simulink model "pendcart_temp"  (Simulink 8.9)
settings: Solver=ode45  StartTime=0.0  StopTime=tsim  RelTol=1e-3  EnableMultiTasking=on
values from neighbouring files (symbols this model uses):
  b = 0.01    [pendcartsim.m]
  c = 0.05    [pendcartsim.m]
  Eta = 0.5882    [pendcartsim.m]
  g = 9.82    [pendcartsim.m]
  K = 0.1    [pendcartsim.m]
  K1 = -119.0071    [pendcartsim.m]
  K2 = 0.0402    [pendcartsim.m]
  l = 0.5    [pendcartsim.m]
  L = 0.001    [pendcartsim.m]
  M = 1    [pendcartsim.m]
  m = 0.5    [pendcartsim.m]
  N = 50    [pendcartsim.m]
  p = 5.4277    [pendcartsim.m]
  p1 = 25.4277    [pendcartsim.m]
  R = 0.6575    [pendcartsim.m]
  theta0 = 5*pi/180    (= 0.0872664625997)    [pendcartsim.m]
  Wheel_Radius = 0.035    [pendcartsim.m]
undefined symbols (not defined in the file or in its folder): Taum, taum
settings Model: Creator=Chris  LastModifiedBy=Administrator
settings OptimizationCC: ExpressionDepthLimit=2147483647  InitFltsAndDblsToZero=on
settings DebuggingCC: AlgebraicLoopMsg=none  SaveWithParameterizedLinksMsg=none
settings GRTTargetCC: TargetFcnLib=ansi_tfl_tmw.mat

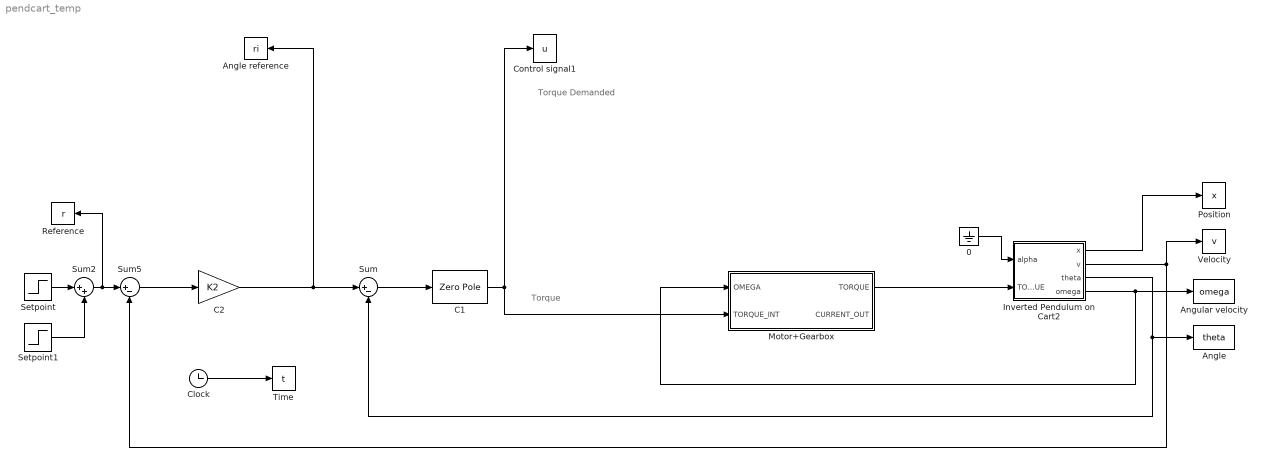
== system pendcart_temp ==
  note: Torque
  note: Torque Demanded
  0 : Ground
  Angle : ToWorkspace  VariableName=theta  SampleTime=-1
  Angle reference : ToWorkspace  VariableName=ri  SampleTime=-1
  Angular velocity : ToWorkspace  VariableName=omega  SampleTime=-1
  C1 : ZeroPole  Zeros=[-p]  Poles=[-p1]  Gain=[K1]
  C2 : Gain  Gain=K2
  Clock : Clock
  Control signal1 : ToWorkspace  VariableName=u  SampleTime=-1
  Inverted Pendulum on Cart2 : Subsystem
  Motor+Gearbox : Subsystem
  Position : ToWorkspace  VariableName=x  SampleTime=-1
  Reference : ToWorkspace  VariableName=r  SampleTime=-1
  Setpoint : Step  Time=10  After=0.5  SampleTime=0
  Setpoint1 : Step  Time=20  After=-0.5  SampleTime=0
  Sum : Sum  Inputs=|+-
  Sum2 : Sum  Inputs=|++
  Sum5 : Sum  Inputs=|+-
  Time : ToWorkspace  VariableName=t  SampleTime=-1
  Velocity : ToWorkspace  VariableName=v  SampleTime=-1
  wires:
  Clock/1 -> Time/1
  Inverted Pendulum on Cart2/1(x) -> Position/1
  Sum/1 -> C1/1
  C1/1 -> Motor+Gearbox/2(TORQUE_INT), Control signal1/1
  Inverted Pendulum on Cart2/2(v) -> Sum5/2, Velocity/1
  Inverted Pendulum on Cart2/3(theta) -> Sum/2, Angle/1
  Sum5/1 -> C2/1
  C2/1 -> Angle reference/1, Sum/1
  Setpoint/1 -> Sum2/1
  Setpoint1/1 -> Sum2/2
  Sum2/1 -> Sum5/1, Reference/1
  0/1 -> Inverted Pendulum on Cart2/1(alpha)
  Inverted Pendulum on Cart2/4(omega) -> Motor+Gearbox/1(OMEGA), Angular velocity/1
  Motor+Gearbox/1(TORQUE) -> Inverted Pendulum on Cart2/2(TORQUE)

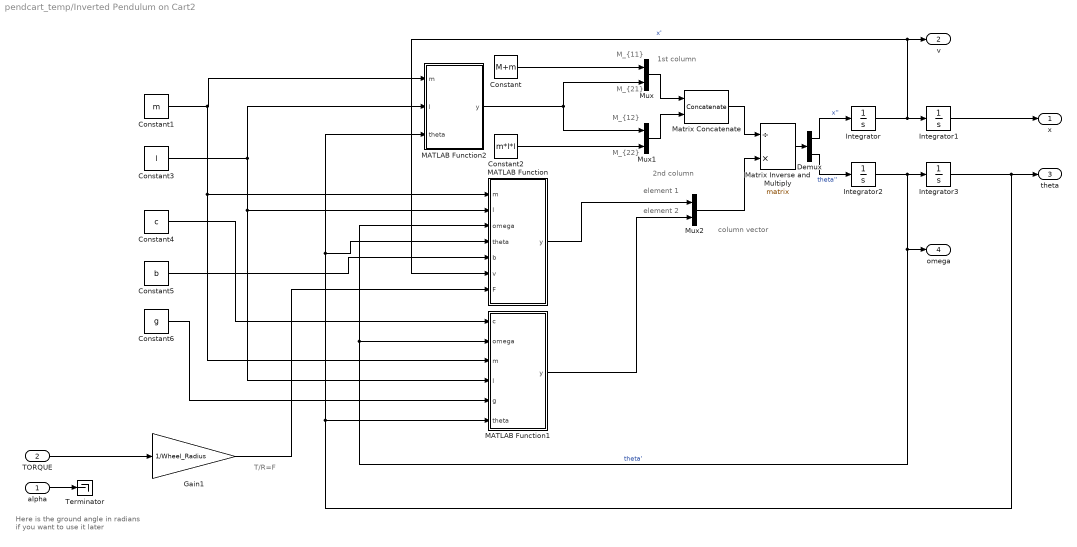
== system pendcart_temp/Inverted Pendulum on Cart2 ==
  note: T/R=F
  note: 2nd column
  note: M_{21}
  note: 1st column
  note: M_{12}
  note: element 2
  note: Here is the ground angle in
      | radians if you want to use it later
  note: column vector
  note: M_{11}
  note: M_{22}
  note: element 1
  alpha : Inport
  TORQUE : Inport  Port=2
  Constant : Constant  Value=M+m
  Constant1 : Constant  Value=m
  Constant2 : Constant  Value=m*l*l
  Constant3 : Constant  Value=l
  Constant4 : Constant  Value=c
  Constant5 : Constant  Value=b
  Constant6 : Constant  Value=g
  Demux : Demux  Outputs=2
  Gain1 : Gain  Gain=1/Wheel_Radius
  Integrator : Integrator
  Integrator1 : Integrator
  Integrator2 : Integrator
  Integrator3 : Integrator  InitialCondition=theta0
  MATLAB Function : MATLAB Function  TreatAsAtomicUnit=on
  MATLAB Function1 : MATLAB Function  TreatAsAtomicUnit=on
  MATLAB Function2 : MATLAB Function  TreatAsAtomicUnit=on
  Matrix Concatenate : Concatenate  Mode=Multidimensional array  ConcatenateDimension=2
  Matrix Inverse and Multiply : Product  Inputs=/*  Multiplication=Matrix(*)
  Mux : Mux  Inputs=2
  Mux1 : Mux  Inputs=2
  Mux2 : Mux  Inputs=2
  Terminator : Terminator
  x : Outport
  v : Outport  Port=2
  theta : Outport  Port=3
  omega : Outport  Port=4
  wires:
  TORQUE/1 -> Gain1/1
  MATLAB Function1/1(y) -> Mux2/2
  Constant1/1 -> MATLAB Function1/3(m), MATLAB Function/1(m), MATLAB Function2/1(m)
  Constant5/1 -> MATLAB Function/5(b)
  Matrix Inverse and Multiply/1 -> Demux/1
  Constant2/1 -> Mux1/2
  Mux2/1 -> Matrix Inverse and Multiply/2
  MATLAB Function/1(y) -> Mux2/1
  Constant4/1 -> MATLAB Function1/1(c)
  Mux1/1 -> Matrix Concatenate/2
  Constant/1 -> Mux/1
  MATLAB Function2/1(y) -> Mux1/1, Mux/2
  Integrator/1 -> Integrator1/1, v/1, MATLAB Function/6(v)  "x'"
  Matrix Concatenate/1 -> Matrix Inverse and Multiply/1
  Integrator1/1 -> x/1
  Demux/2 -> Integrator2/1  "theta''"
  Integrator3/1 -> MATLAB Function/4(theta), MATLAB Function2/3(theta), MATLAB Function1/6(theta), theta/1
  Constant3/1 -> MATLAB Function1/4(l), MATLAB Function/2(l), MATLAB Function2/2(l)
  Mux/1 -> Matrix Concatenate/1
  Integrator2/1 -> Integrator3/1, MATLAB Function/3(omega), MATLAB Function1/2(omega), omega/1  "theta'"
  Constant6/1 -> MATLAB Function1/5(g)
  alpha/1 -> Terminator/1
  Demux/1 -> Integrator/1  "x''"
  Gain1/1 -> MATLAB Function/7(F)

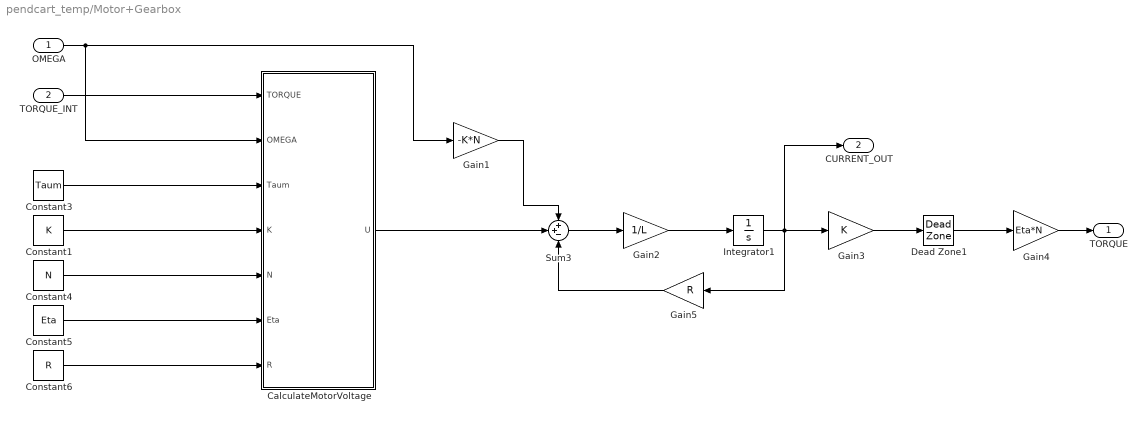
== system pendcart_temp/Motor+Gearbox ==
  OMEGA : Inport
  TORQUE_INT : Inport  Port=2
  CalculateMotorVoltage : MATLAB Function  TreatAsAtomicUnit=on
  Constant1 : Constant  Value=K
  Constant3 : Constant  Value=Taum
  Constant4 : Constant  Value=N
  Constant5 : Constant  Value=Eta
  Constant6 : Constant  Value=R
  Dead Zone1 : DeadZone  LowerValue=-taum  UpperValue=taum  SaturateOnIntegerOverflow=on
  Gain1 : Gain  Gain=-K*N
  Gain2 : Gain  Gain=1/L
  Gain3 : Gain  Gain=K
  Gain4 : Gain  Gain=Eta*N
  Gain5 : Gain  Gain=R
  Integrator1 : Integrator
  Sum3 : Sum  Inputs=++-
  TORQUE : Outport
  "CURRENT_OUT " : Outport  Port=2
  wires:
  OMEGA/1 -> CalculateMotorVoltage/2(OMEGA), Gain1/1
  Integrator1/1 -> "CURRENT_OUT "/1, Gain5/1, Gain3/1
  Sum3/1 -> Gain2/1
  Gain5/1 -> Sum3/3
  CalculateMotorVoltage/1(U) -> Sum3/2
  Gain1/1 -> Sum3/1
  Gain2/1 -> Integrator1/1
  Gain3/1 -> Dead Zone1/1
  Gain4/1 -> TORQUE/1
  Dead Zone1/1 -> Gain4/1
  Constant1/1 -> CalculateMotorVoltage/4(K)
  Constant3/1 -> CalculateMotorVoltage/3(Taum)
  Constant4/1 -> CalculateMotorVoltage/5(N)
  Constant5/1 -> CalculateMotorVoltage/6(Eta)
  Constant6/1 -> CalculateMotorVoltage/7(R)
  TORQUE_INT/1 -> CalculateMotorVoltage/1(TORQUE)

== matlab function Inverted Pendulum on Cart2/MATLAB Function1 ==
  data: y output double; c input double; omega input double; m input double; l input double; g input double; theta input double
function y  = fcn(c,omega,m,l,g,theta)

y =c*omega+m*l*g*sin(theta);

== matlab function Inverted Pendulum on Cart2/MATLAB Function ==
  data: y output double; m input double; l input double; omega input double; theta input double; b input double; v input double; F input double
function y = fcn(m,l,omega,theta,b,v,F)

y =m*l*omega*omega*sin(theta)+b*v+F;

== matlab function Inverted Pendulum on Cart2/MATLAB Function2 ==
  data: y output double; m input double; l input double; theta input double
function y = fcn(m,l,theta)

y =m*l*cos(theta);

== matlab function Motor+Gearbox/CalculateMotorVoltage ==
  data: U output double; TORQUE input double; OMEGA input double; Taum input double; K input double; N input double; Eta input double; R input double
function U  = CalculateMotorVoltage(TORQUE,OMEGA,Taum,K,N,Eta,R)
%CALCULATEMOTORVOLTAGE Summary of this function goes here
%   Detailed explanation goes here
   
    if T == 0
        i = 0;
    else
        if T>0
			 i = TORQUE/(Eta*N*K)+Taum/K;
        else
			 i = TORQUE/(Eta*N*K)-Taum/K;
        end
    end
    U = R*i + N*K*OMEGA;
end
